simulink model "mrac_filter"  (R2023a)
settings: Solver=ode5  StartTime=0.0  StopTime=120  FixedStep=0.001  RelTol=1e-3
settings Model: Creator=merve  LastModifiedBy=merve
settings DataIOCC: ReturnWorkspaceOutputs=off

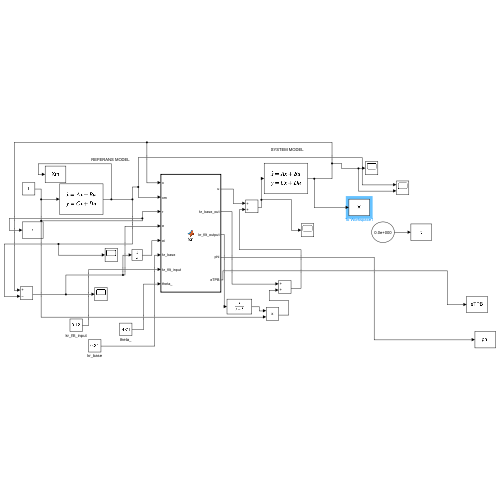
[thumbnail: Simulink's stored preview of the top-level diagram]
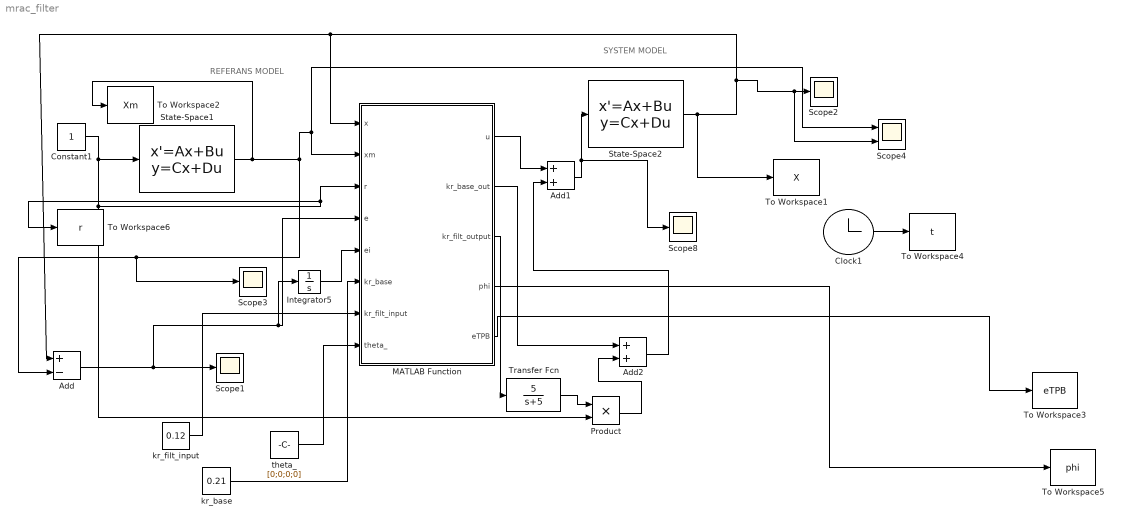
== system mrac_filter ==
  note: REFERANS MODEL
  note: SYSTEM MODEL
  Add : Sum  Inputs=+-
  Add1 : Sum
  Add2 : Sum
  Clock1 : Clock
  Constant1 : Constant  SampleTime=-1
  Integrator5 : Integrator
  MATLAB Function : MATLAB Function  TreatAsAtomicUnit=on
  Product : Product
  Scope{1..3,8} (4 alike) : Scope
  Scope4 : Scope  NumInputPorts=2
  State-Space1 : StateSpace  A=[0 1;-0.23 -0.71]  B=[0;0.23]  C=[1 0;0 1]  D=[0;0]  InitialCondition=0
  State-Space2 : StateSpace  A=[-0.0714 61;-1 -300]  B=[0;10]  C=[1 0;0 1]  D=[0;0]  InitialCondition=0
  To Workspace1 : ToWorkspace  VariableName=X  SaveFormat=Structure With Time  SampleTime=-1
  To Workspace2 : ToWorkspace  VariableName=Xm  SaveFormat=Structure With Time  SampleTime=-1
  To Workspace3 : ToWorkspace  VariableName=eTPB  SaveFormat=Structure With Time  SampleTime=-1
  To Workspace4 : ToWorkspace  VariableName=t  SaveFormat=Structure With Time  SampleTime=-1
  To Workspace5 : ToWorkspace  VariableName=phi  SaveFormat=Structure With Time  SampleTime=-1
  To Workspace6 : ToWorkspace  VariableName=r  SaveFormat=Structure With Time  SampleTime=-1
  Transfer Fcn : TransferFcn  Numerator=[5]  Denominator=[1 5]
  kr_base : Constant  Value=0.21  SampleTime=-1
  kr_filt_input : Constant  Value=0.12  SampleTime=-1
  theta_ : Constant  Value=[0;0;0;0]  VectorParams1D=off  SampleTime=-1
  wires:
  Constant1/1 -> State-Space1/1, To Workspace6/1, MATLAB Function/3(r), Product/2
  State-Space2/1 -> To Workspace1/1, Scope4/2, Scope2/1, MATLAB Function/1(x), Add/1
  Add/1 -> Integrator5/1, MATLAB Function/4(e), Scope1/1
  MATLAB Function/1(u) -> Add1/1
  Clock1/1 -> To Workspace4/1
  State-Space1/1 -> To Workspace2/1, Scope4/1, MATLAB Function/2(xm), Scope3/1, Add/2
  Integrator5/1 -> MATLAB Function/5(ei)
  MATLAB Function/2(kr_base_out) -> Add2/1
  MATLAB Function/3(kr_filt_output) -> Transfer Fcn/1
  Transfer Fcn/1 -> Product/1
  Product/1 -> Add2/2
  Add2/1 -> Add1/2
  Add1/1 -> State-Space2/1, Scope8/1
  kr_base/1 -> MATLAB Function/6(kr_base)
  kr_filt_input/1 -> MATLAB Function/7(kr_filt_input)
  theta_/1 -> MATLAB Function/8(theta_)
  MATLAB Function/4(phi) -> To Workspace5/1
  MATLAB Function/5(eTPB) -> To Workspace3/1

== matlab function mrac_filter/MATLAB Function ==
  settings: updateMethod=DISCRETE
  data: x input; u output; xm input; r input; e input; ei input; kr_base_out output; kr_filt_output output; phi output; eTPB output; kr_base input; kr_filt_input input; theta_ input
function [u, kr_base_out, kr_filt_output,phi,eTPB] = fcn(x, xm, r, e, ei,kr_base,kr_filt_input,theta_)

    

    P = [2.799 3.125; 3.125 6.359];
    B = [0; 1];

    phi = [x; ei];
    eTPB = e' * P * B;

   kr_base_out=kr_base;
   kr_filt_output=kr_filt_input;
    Kr = [-0.16; -0.57];
    % Kontrol sinyali
    % kr = kr_base + kr_filt_output → bu hesap Simulink'te yapılmalı
    % (yani Transfer Fcn bloğuyla)
    u = Kr' * x + theta_' * phi;

end
